simulink model "ContainerVesselPIDspeedControl"  (R2022a)
settings: Solver=ode4  StartTime=0.0  StopTime=600  FixedStep=0.1  RelTol=1e-3  EnableMultiTasking=on
libraries: simulink x2, simulink_need_slupdate x1, slpidlib x1
settings Model: Creator=hntran  LastModifiedBy=hntran
settings DataIOCC: ReturnWorkspaceOutputs=off

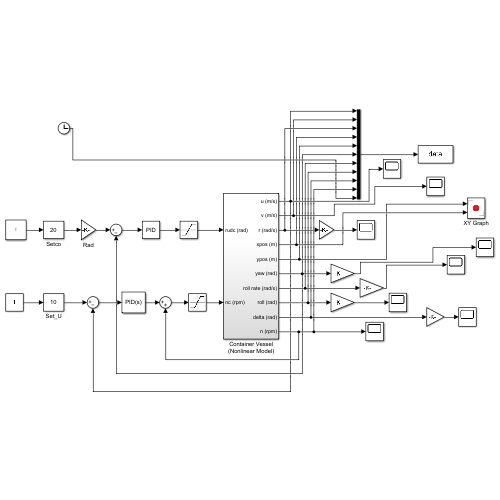
[thumbnail: Simulink's stored preview of the top-level diagram]
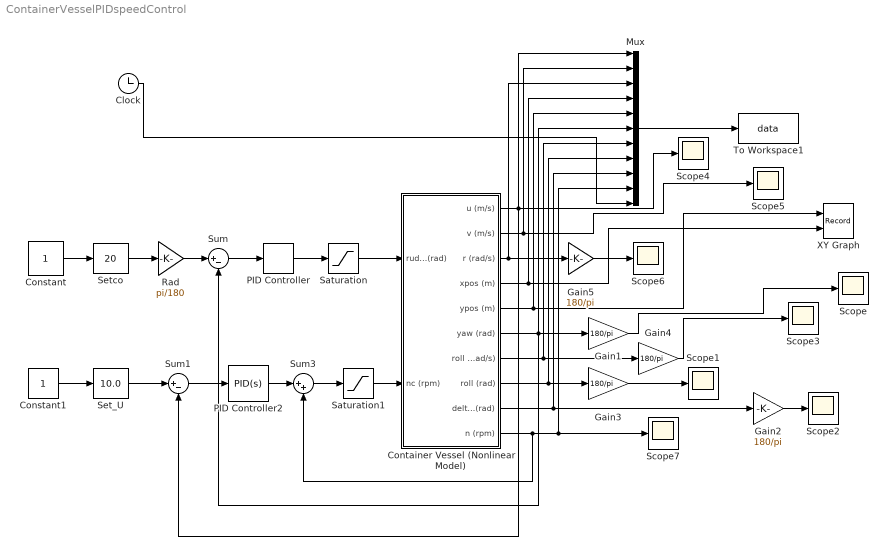
== system ContainerVesselPIDspeedControl ==
  Clock : Clock
  Constant : Constant
  Constant1 : Constant
  Container Vessel (Nonlinear Model) : Subsystem
  Gain{1..5} (5 alike) : Gain  Gain=180/pi
  Mux : Mux  Inputs=11
  PID Controller : simulink_need_slupdate/PID Controller  P=5  I=0.0025  D=20
  PID Controller2 : slpidlib/PID Controller  Controller=PID  Form=Parallel  TimeDomain=Continuous-time  UseExternalTs=off  SampleTime=-1  IntegratorMethod=Forward Euler  FilterMethod=Forward Euler  ControllerParametersSource=internal  P=196.032112345719  I=5.90037217771751  UseKiTs=off  D=414.381346752507  N=20.1381355803379  UseFilter=on  TunerSelectOption=Transfer Function Based (PID Tuner App)  InitialConditionSource=internal  InitialConditionForIntegrator=0  InitialConditionForFilter=0  DifferentiatorICPrevScaledInput=0  ExternalReset=none  TrackingMode=off  Kt=1  LimitOutput=off  SatLimitsSource=internal  UpperSaturationLimit=inf  LowerSaturationLimit=-inf  LinearizeAsGain=on  AntiWindupMode=none  Kb=1  POutMin=[]  POutMax=[]  IOutMin=[]  IOutMax=[]  DOutMin=[]  DOutMax=[]  NOutMin=[]  NOutMax=[]  SumOutMin=[]  SumOutMax=[]  SaturationOutMin=[]  SaturationOutMax=[]  PParamMin=[]  PParamMax=[]  IParamMin=[]  IParamMax=[]  DParamMin=[]  DParamMax=[]  NParamMin=[]  NParamMax=[]  KbParamMin=[]  KbParamMax=[]  KtParamMin=[]  KtParamMax=[]  KbOutMin=[]  KbOutMax=[]  KtOutMin=[]  KtOutMax=[]  IntegratorOutMin=[]  IntegratorOutMax=[]  FilterOutMin=[]  FilterOutMax=[]  SumI1OutMin=[]  SumI1OutMax=[]  SumI2OutMin=[]  SumI2OutMax=[]  SumI3OutMin=[]  SumI3OutMax=[]  SumI4OutMin=[]  SumI4OutMax=[]  SumDOutMin=[]  SumDOutMax=[]  DifferentiatorOutMin=[]  DifferentiatorOutMax=[]  FilterDiffOutCoefMin=[]  FilterDiffOutCoefMax=[]  ReciprocalOutMin=[]  ReciprocalOutMax=[]  SumDenOutMin=[]  SumDenOutMax=[]  SumNumOutMin=[]  SumNumOutMax=[]  DivideOutMin=[]  DivideOutMax=[]  UdiffTsProdOutMin=[]  UdiffTsProdOutMax=[]  NTsProdOutMin=[]  NTsProdOutMax=[]  UintegralTsProdOutMin=[]  UintegralTsProdOutMax=[]  UngainTsProdOutMin=[]  UngainTsProdOutMax=[]  IntegratorContinuousStateAttributes=''  IntegratorStateMustResolveToSignalObject=off  IntegratorRTWStateStorageClass=Auto  FilterContinuousStateAttributes=''  FilterStateMustResolveToSignalObject=off  FilterRTWStateStorageClass=Auto  ParallelPVariant=InternalParameters  IdealPVariant=Disabled  IVariant=InternalParameters  DVariant=InternalParameters  IntegratorVariant=Continuous  SatVariant=Disabled  AWVariant=Passthrough  PCopyVariant=Disabled  TRVariant=Disabled  FdbkBlocksVariant=Forward  IdealPFdbkVariant=Disabled  SatFdbkVariant=Disabled  DerivativeFilterVariant=ContFilter  NVariant=InternalParameters  NCopyVariant=Disabled  FilterICVariant=InternalICsFilter  IntegratorICVariant=InternalICs  ExternalResetVariant=Disabled  TRSumVariant=Passthrough  SumFdbkVariant=Disabled  SumVariant=Sum_PID  TsampFilterVariant=InternalTs  TsampNgainVariant=Passthrough  TsampIntegralVariant=Passthrough  ExternalSaturationOutDataTypeStr=Inherit: Same as second input  aMode=0
  Rad : Gain  Gain=pi/180  SaturateOnIntegerOverflow=on  OutDataTypeStr=Inherit: Same as input  ParamDataTypeStr=Inherit: Same as input
  Saturation : Saturate  UpperLimit=10*pi/180  LowerLimit=-10*pi/180
  Saturation1 : Saturate  UpperLimit=200  LowerLimit=1
  Scope{,1..7} (8 alike) : Scope
  Set_U : simulink/Math Operations/Slider Gain  gain=10.0  low=1  high=10
  Setco : simulink/Math Operations/Slider Gain  gain=20  low=0  high=360
  Sum : Sum  Inputs=|+-
  Sum1 : Sum  Inputs=|+-
  Sum3 : Sum  Inputs=|++
  To Workspace1 : ToWorkspace  VariableName=data  SampleTime=-1
      settings: Decimation=2
  XY Graph : Record  FileSettingsInternal="{\"entries\":[{\"content\":{\"excelSettings\":{\"content\":{},\"type\":\"Streamout.ExcelSettings\"}},\"type\":\"Streamout.FileSettingStorage\",\"uuid\":\"ed4bb2cf-d8da-49ff-9710-cf5ea79b5470\"}],\"packageUris\":[\"http://schema.mathworks.com/mf0/streamout_blocks/R2020a\"],\"version\":\"1.0\"}"  Layout=[1 1]  SignalsInternal="{\"entries\":[{\"content\":{\"signals\":[{\"content\":{\"blockPath\":[\"ContainerVesselPIDspeedControl/XY Graph\"],\"channel\":[],\"dimensions\":[1],\"domain\":\"ContainerVesselPIDspeedControl/XY Graph\",\"lineColor\":\"#a2142f\",\"plots\":[1],\"port\":1,\"sid\":[\"\"],\"signalID\":3284,\"signalName\":\"Container Vessel\\n(Nonlinear Model):5\"},\"type\":\"RecordBlkView.Signal\",\"uuid\":\"d79fec90-6445-4035-8097-5b2f5eabe7ed\"},{\"content\":{\"blockPath\":[\"ContainerVesselPIDspeedControl/XY Graph\"],\"channel\":[],\"dimensions\":[1],\"domain\":\"ContainerVesselPIDspeedControl/XY Graph\",\"lineColor\":\"#139fff\",\"plots\":[1],\"port\":2,\"sid\":[\"\"],\"signalID\":3288,\"signalName\":\"Container Vessel\\n(Nonlinear Model):4\"},\"type\":\"RecordBlkView.Signal\",\"uuid\":\"16dae710-454e-413f-a461-a4a1fdee4adc\"}]},\"type\":\"RecordBlkView.InputSignals\",\"uuid\":\"8ba0d1ba-b029-4a36-8825-5099d8635969\"}],\"packageUris\":[\"http://schema.mathworks.com/mf0/streamout_blocks/R2020a\"],\"version\":\"1.0\"}"  VisualizationBindings="{\"xyplotplugin\":{\"info\":[{\"series\":[{\"bindingParametersList\":[{\"parameter\":\"X-Axis\",\"signalID\":3284,\"signalName\":\"Container Vessel\\n(Nonlinear Model):5\"},{\"parameter\":\"Y-Axis\",\"signalID\":3288,\"signalName\":\"Container Vessel\\n(Nonlinear Model):4\"}],\"seriesID\":19158}],\"subplotID\":1}]}}"  CompatibilityTag=XY  st=-1
  wires:
  Container Vessel (Nonlinear Model)/8(roll (rad)) -> Gain3/1, Mux/8
  Gain5/1 -> Scope6/1
  Container Vessel (Nonlinear Model)/7(roll rate (rad/s)) -> Mux/7, Gain4/1
  Mux/1 -> To Workspace1/1
  Gain2/1 -> Scope2/1
  Container Vessel (Nonlinear Model)/1(u (m/s)) -> Sum1/2, Scope4/1, Mux/1
  Container Vessel (Nonlinear Model)/4(xpos (m)) -> XY Graph/2, Mux/4
  Container Vessel (Nonlinear Model)/5(ypos (m)) -> XY Graph/1, Mux/5
  Container Vessel (Nonlinear Model)/3(r (rad/s)) -> Gain5/1, Mux/3
  Gain4/1 -> Scope3/1
  Container Vessel (Nonlinear Model)/6(yaw (rad)) -> Sum/2, Gain1/1, Mux/6
  Gain1/1 -> Scope/1
  Container Vessel (Nonlinear Model)/2(v (m/s)) -> Scope5/1, Mux/2
  Container Vessel (Nonlinear Model)/10(n (rpm)) -> Sum3/2, Scope7/1, Mux/10
  Gain3/1 -> Scope1/1
  Container Vessel (Nonlinear Model)/9(delta (rad)) -> Gain2/1, Mux/9
  Clock/1 -> Mux/11
  Constant1/1 -> Set_U/1
  Set_U/1 -> Sum1/1
  Saturation1/1 -> Container Vessel (Nonlinear Model)/2(nc (rpm))
  Sum3/1 -> Saturation1/1
  Sum/1 -> PID Controller/1
  Setco/1 -> Rad/1
  Rad/1 -> Sum/1
  PID Controller/1 -> Saturation/1
  Constant/1 -> Setco/1
  Saturation/1 -> Container Vessel (Nonlinear Model)/1(rudc (rad))
  Sum1/1 -> PID Controller2/1
  PID Controller2/1 -> Sum3/1

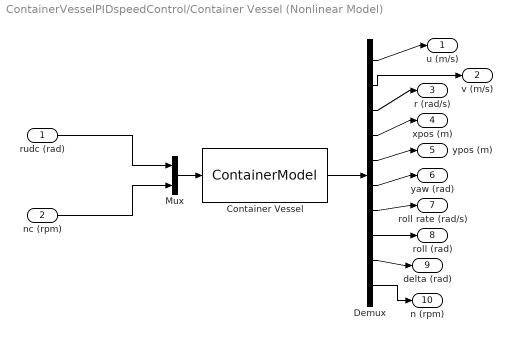
== system ContainerVesselPIDspeedControl/Container Vessel (Nonlinear Model) ==
  rudc (rad) : Inport
  nc (rpm) : Inport  Port=2
  Container Vessel : S-Function  FunctionName=ContainerModel  SFunctionDeploymentMode=off  EnableBusSupport=off
  Demux : Demux  Outputs=10
  Mux : Mux  Inputs=2
  u (m/s) : Outport
  v (m/s) : Outport  Port=2
  r (rad/s) : Outport  Port=3
  xpos (m) : Outport  Port=4
  ypos (m) : Outport  Port=5
  yaw (rad) : Outport  Port=6
  roll rate (rad/s) : Outport  Port=7
  roll (rad) : Outport  Port=8
  delta (rad) : Outport  Port=9
  n (rpm) : Outport  Port=10
  wires:
  Mux/1 -> Container Vessel/1
  Container Vessel/1 -> Demux/1
  Demux/1 -> u (m/s)/1
  Demux/2 -> v (m/s)/1
  Demux/3 -> r (rad/s)/1
  Demux/4 -> xpos (m)/1
  Demux/5 -> ypos (m)/1
  Demux/6 -> yaw (rad)/1
  nc (rpm)/1 -> Mux/2
  Demux/7 -> roll rate (rad/s)/1
  Demux/8 -> roll (rad)/1
  Demux/9 -> delta (rad)/1
  Demux/10 -> n (rpm)/1
  rudc (rad)/1 -> Mux/1
